simulink subsystem "Shrimple_6dof_parachute"  (R2025a)
settings: Solver=VariableStepAuto  StartTime=0.0  StopTime=10.0  RelTol=1e-3
undefined symbols (not defined in the file): Apogee_stop, BG0, Burnout_stop, COM_table, F, HG0, I, ignition_delay, include_turbulence, latlong0, launch_elevation, Light, m_table, MIL, MOI_table, time0, turbulence_noise_seeds, uvw0_B, v0_NED, w0_BN, x0_NED
libraries: sharedtransform x2, aerolibwind2 x1
settings Model: Creator=thatf  LastModifiedBy=thatf
settings RTWCC: GPUComputeCapability=3.5

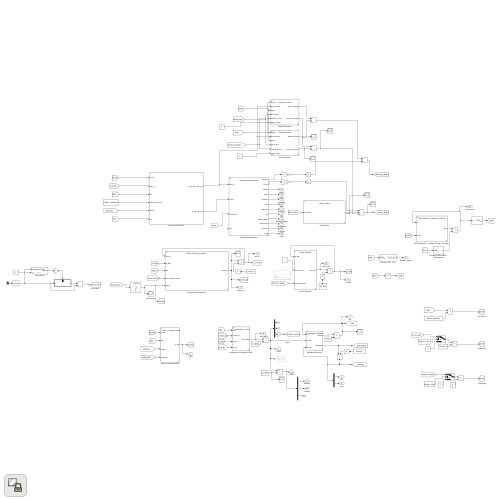
[thumbnail: Simulink's stored preview of the top-level diagram]
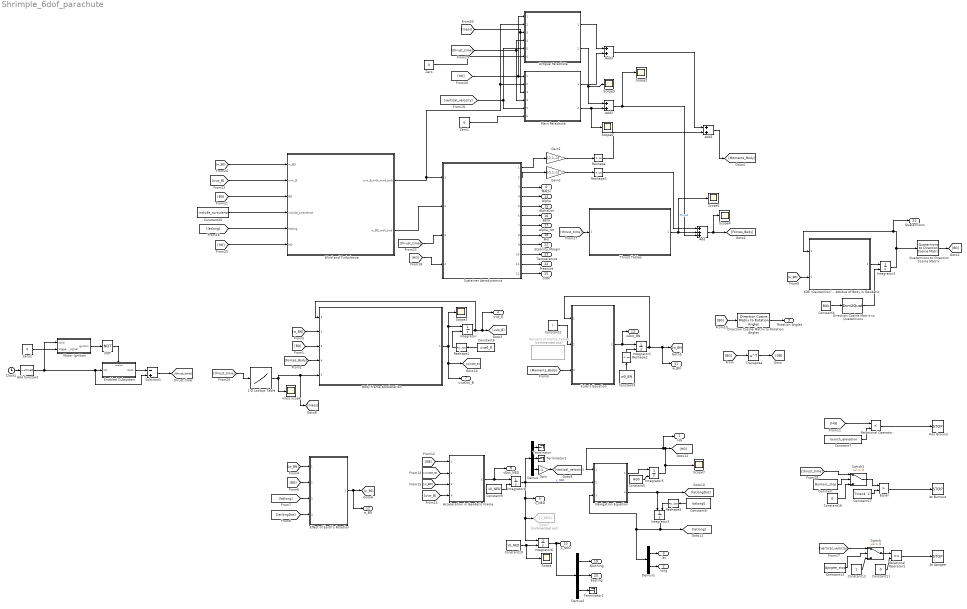
== system Shrimple_6dof_parachute ==
  1-D Lookup Table : Lookup_n-D  NumberOfTableDimensions=1  BreakpointsForDimension1=m_table(:,1)  Table=m_table(:,2)  InternalRulePriority=Speed  RndMeth=Simplest
  Acceleration in Geodetic Frame : Subsystem  ReferencedSubsystem=Acceleration_in_Geodetic_Frame
  Add : Sum  Inputs=+++
  Add Constant : Bias  Bias=time0  SaturateOnIntegerOverflow=off
  Add1 : Sum
  Add2 : Sum
  Add3 : Sum
  At Apogee : Stop
  At Burnout : Stop
  Body Frame Acceleration : Subsystem  ReferencedSubsystem=Body_Frame_Acceleration
  Clock1 : Clock
  Constant : Constant  Value=Burnout_stop
  Constant10 : Constant  Value=x0_NED
  Constant11 : Constant  Value=0
  Constant12 : Constant
  Constant13 : Constant  Value=Apogee_stop
  Constant16 : Constant  Value=0
  Constant17 : Constant  Value=Tx(end, 1)
  Constant2 : Constant  Value=I
  Constant20 : Constant  Value=include_turbulence
  Constant3 : Constant  Value=w0_BN
  Constant4 : Constant  Value=BG0
  Constant5 : Constant  Value=HG0
  Constant6 : Constant  Value=uvw0_B
  Constant7 : Constant  Value=launch_elevation
  Constant8 : Constant  Value=latlong0
  Constant9 : Constant  Value=v0_NED
  Demux : Demux  Outputs=3
  Demux1 : Demux  Outputs=2
  Demux2 : Demux  Outputs=3
  Direction Cosine Matrix to Rotation Angles : sharedtransform/Direction Cosine Matrix to Rotation Angles  rotationOrder=ZYX  aMode=aMode  action=None  tolerance=eps(2)
  Direction Cosine Matrix to Quaternions : Dcm2Quat
  Drogue Parachute : Subsystem  ReferencedSubsystem=Parachute_model  radius=drogue_radius  Cd=drogue_CD  parachute_deployment_type=ParachuteDeploymentType.Apogee_Delay_Deployment  burnout_delay=0  deploy_height=0
  Effect of Earth's Rotation : Subsystem  ReferencedSubsystem=Effect_of_Earths_Rotation
  Enabled Subsystem : Subsystem  TreatAsAtomicUnit=on
  Equal : RelationalOperator  Operator=>  OutDataTypeStr=boolean  RndMeth=Simplest  InputSameDT=off
  Euler's Equation : Subsystem  ReferencedSubsystem=Eulers_Equation
  Gain : Gain  Gain=-1
  Gain1 : Gain  Gain=[-1,1,-1]
  Gain2 : Gain  Gain=[-1,1,-1]
  Goto7 : Goto  Commented=on  GotoTag=v_NED
  Hits Ground : Stop
  Integrator{,1..6} (7 alike) : Integrator  InitialConditionSource=external
  "KDE (Qauternion) -  Attidue of Body in Geodetic " : Subsystem  ReferencedSubsystem=KDE_Qauternion_Attitude_of_Body_in_Geodetic
  Main Parachute : Subsystem  ReferencedSubsystem=Parachute_model  radius=main_radius  Cd=main_CD  parachute_deployment_type=ParachuteDeploymentType.Elevation_Deployment  burnout_delay=0  deploy_height=300
  Moment of Inertia Tables : Subsystem  Commented=on
  Motor Ignition : Subsystem  Variant=on
  NOT : Logic  Operator=NOT  IconShape=distinctive  AllPortsSameDT=off  OutDataTypeStr=boolean
  Navigation Equation : Subsystem  ReferencedSubsystem=Navigation_Equation
  Quaternions to Direction Cosine Matrix : sharedtransform/Quaternions to  Direction Cosine Matrix  aMode=aMode
  Relational Operator : RelationalOperator  Operator=<  OutDataTypeStr=boolean  RndMeth=Simplest  InputSameDT=off
  Relational Operator1 : RelationalOperator  Operator=<=  OutDataTypeStr=boolean  RndMeth=Simplest  InputSameDT=off
  Reshape{,1..3} (4 alike) : Reshape  OutputDimensionality=Customize  OutputDimensions=[3,1]
  Reshape4 : Reshape  OutputDimensionality=Customize  OutputDimensions=[2,1]
  Scope{,1..7} (8 alike) : Scope
      Scope settings: ActiveDisplayYMinimum=-435.13988  ActiveDisplayYMaximum=48.34887  DataLoggingVariableName=ScopeData11
      Scope1 settings: ActiveDisplayYMinimum=-123.17299  ActiveDisplayYMaximum=58.34227  DataLoggingVariableName=ScopeData12
      Scope2 settings: ActiveDisplayYMinimum=-1  ActiveDisplayYMaximum=1  DataLoggingVariableName=ScopeData13
      Scope3 settings: ActiveDisplayYMinimum=-153.18625  ActiveDisplayYMaximum=463.92065  DataLoggingVariableName=ScopeData14
      Scope4 settings: ActiveDisplayYMinimum=-123.17299  ActiveDisplayYMaximum=58.34227  DataLoggingVariableName=ScopeData15
      Scope5 settings: ActiveDisplayYMinimum=-1  ActiveDisplayYMaximum=1  DataLoggingVariableName=ScopeData7
      Scope6 settings: ActiveDisplayYMinimum=-1  ActiveDisplayYMaximum=1  DataLoggingVariableName=ScopeData8
      Scope7 settings: ActiveDisplayYMinimum=-1765.05046  ActiveDisplayYMaximum=15985.4541  DataLoggingVariableName=ScopeData16
  Subtract1 : Sum  Inputs=-+
  Sustainer Aerodynamics : Subsystem  ReferencedSubsystem=Sustainer_Aerodynamics
  Switch : Switch  Criteria=u2 > Threshold  SaturateOnIntegerOverflow=off  InputSameDT=off
  Switch1 : Switch  Criteria=u2 > Threshold  SaturateOnIntegerOverflow=off  InputSameDT=off
  Terminator : Terminator
  Terminator1 : Terminator
  Terminator2 : Terminator
  Thrust Tables : Subsystem  ReferencedSubsystem=Thrust_Tables
  Transpose : Math  Operator=transpose
  Wind and Turbulence : Subsystem
  Zero : Constant  Value=0  OutDataTypeStr=Inherit: Inherit via back propagation
  Zero1 : Constant  Value=0  OutDataTypeStr=Inherit: Inherit via back propagation
  Zero2 : Constant  Value=0  OutDataTypeStr=Inherit: Inherit via back propagation
  mass scope : Scope
      settings: ActiveDisplayYMinimum=12.9015  ActiveDisplayYMaximum=24.17549  DataLoggingVariableName=ScopeData17
  HG : Outport
  long : Outport  Port=2
  lat : Outport  Port=3
  uvw_B : Outport  Port=4
  v_NED : Outport  Port=5
  MACH : Outport  Port=6
  uvwDot_B : Outport  Port=7
  vDot_NED : Outport  Port=8
  Rotation Angles : Outport  Port=9
  x_NED : Outport  Port=10
  w_BN : Outport  Port=11
  w_BG : Outport  Port=12
  wDot_BN : Outport  Port=13
  Alpha : Outport  Port=14
  AlphaDot : Outport  Port=15
  Beta : Outport  Port=16
  Alpha_tot : Outport  Port=17
  PHI : Outport  Port=18
  Northing : Outport  Port=19
  Easting : Outport  Port=20
  Quaternions : Outport  Port=21
  Stability_Margin : Outport  Port=22
  Temperature : Outport  Port=23
  Pressure : Outport  Port=24
  COM : Outport  Port=25
  wires:
  Euler's Equation/1 -> Integrator1/1, wDot_BN/1
  Direction Cosine Matrix to Rotation Angles/1 -> Rotation Angles/1
  [BG] -> Direction Cosine Matrix to Rotation Angles/1
  Direction Cosine Matrix to Quaternions/1 -> Integrator2/2
  Constant5/1 -> Integrator5/2
  [BG] -> Transpose/1
  [BG] -> Body Frame Acceleration/3
  [w_BG] -> Acceleration in Geodetic Frame/3
  Reshape/1 -> Add1/2
  Constant6/1 -> Reshape1/1
  Navigation Equation/2 -> Integrator3/1, [latlongDot]
  Integrator2/1 -> Quaternions to Direction Cosine Matrix/1, "KDE (Qauternion) -  Attidue of Body in Geodetic "/1, Quaternions/1
  Constant3/1 -> Reshape2/1
  [BG] -> Effect of Earth's Rotation/2
  [uvw_B] -> Acceleration in Geodetic Frame/4
  [w_BG] -> "KDE (Qauternion) -  Attidue of Body in Geodetic "/2
  Reshape2/1 -> Integrator1/2
  Reshape1/1 -> Integrator/2
  Integrator3/1 -> Navigation Equation/3, Demux1/1, [latlong]
  Acceleration in Geodetic Frame/1 -> Integrator4/1, vDot_NED/1
  Body Frame Acceleration/1 -> Integrator/1, Scope3/1, [uvwDot_B], uvwDot_B/1
  Navigation Equation/1 -> Integrator5/1
  Constant4/1 -> Direction Cosine Matrix to Quaternions/1
  Integrator5/1 -> [HG], HG/1, Navigation Equation/1, Scope7/1
  "KDE (Qauternion) -  Attidue of Body in Geodetic "/1 -> Integrator2/1
  [Moments_Body] -> Euler's Equation/3
  [w_BN] -> Effect of Earth's Rotation/1
  Integrator4/1 -> v_NED/1, Goto7/1, Integrator6/1, Navigation Equation/2, Demux/1  "v_NED"
  [w_BN] -> Body Frame Acceleration/2
  Integrator/1 -> Body Frame Acceleration/1, [uvw_B], uvw_B/1
  Quaternions to Direction Cosine Matrix/1 -> [BG]
  [uvwDot_B] -> Acceleration in Geodetic Frame/2
  Effect of Earth's Rotation/1 -> [w_BG], w_BG/1
  [GB] -> Acceleration in Geodetic Frame/1
  Transpose/1 -> [GB]
  Relational Operator/1 -> Hits Ground/1
  [Forces_Body] -> Body Frame Acceleration/4
  [latlongDot] -> Effect of Earth's Rotation/4
  Constant7/1 -> Relational Operator/2
  [latlong] -> Effect of Earth's Rotation/3
  Constant9/1 -> Integrator4/2
  Reshape4/1 -> Integrator3/2
  Integrator1/1 -> Euler's Equation/1, [w_BN], w_BN/1
  Constant8/1 -> Reshape4/1
  Demux1/2 -> long/1
  Demux1/1 -> lat/1
  Constant10/1 -> Integrator6/2, Scope/1
  Integrator6/1 -> x_NED/1, Demux2/1
  Reshape3/1 -> Add/1
  Thrust Tables/1 -> Add/2, Scope1/1  "Thrust"
  Add/1 -> [Forces_Body], Scope4/1
  1-D Lookup Table/1 -> Body Frame Acceleration/5, [mass], mass scope/1
  Gain1/1 -> Reshape/1
  Gain2/1 -> Reshape3/1
  Demux2/3 -> Terminator2/1
  Sustainer Aerodynamics/8 -> PHI/1
  Sustainer Aerodynamics/7 -> Alpha_tot/1
  Sustainer Aerodynamics/6 -> Beta/1
  Sustainer Aerodynamics/5 -> AlphaDot/1
  Sustainer Aerodynamics/4 -> Alpha/1
  Sustainer Aerodynamics/3 -> MACH/1
  Sustainer Aerodynamics/2 -> Gain2/1
  Sustainer Aerodynamics/1 -> Gain1/1
  [HG] -> Sustainer Aerodynamics/4
  Sustainer Aerodynamics/9 -> Stability_Margin/1
  Equal/1 -> At Burnout/1
  Constant/1 -> Switch1/2
  Constant16/1 -> Switch1/3
  Constant17/1 -> Equal/2
  Switch1/1 -> Equal/1
  [thrust_time] -> Switch1/1
  Constant2/1 -> Euler's Equation/2
  Demux2/1 -> Northing/1
  Demux2/2 -> Easting/1
  [w_BG] -> Wind and Turbulence/1(w_BG)
  [uvw_B] -> Wind and Turbulence/2(uvw_B)
  [BG] -> Wind and Turbulence/3(BG)
  Constant20/1 -> Wind and Turbulence/4(include_turbulence)
  [latlong] -> Wind and Turbulence/5(latlong)
  [HG] -> Wind and Turbulence/6(HG)
  Wind and Turbulence/1(uvw_B_with_wind_turb) -> Sustainer Aerodynamics/1, Main Parachute/2, Drogue Parachute/2
  Wind and Turbulence/2(w_BG_with_turb) -> Sustainer Aerodynamics/2
  [HG] -> Relational Operator/1
  Constant13/1 -> Switch/2
  Constant12/1 -> Switch/3
  Switch/1 -> Relational Operator1/1
  Constant11/1 -> Relational Operator1/2
  Relational Operator1/1 -> At Apogee/1
  [HG] -> Main Parachute/1, Drogue Parachute/1
  [vertical_velocity] -> Drogue Parachute/5, Main Parachute/5
  Add1/1 -> [Moments_Body]
  Sustainer Aerodynamics/10 -> Temperature/1
  Sustainer Aerodynamics/11 -> Pressure/1
  Subtract1/1 -> [thrust_time]
  [thrust_time] -> 1-D Lookup Table/1
  [thrust_time] -> Thrust Tables/1
  Clock1/1 -> Add Constant/1
  Add Constant/1 -> Enabled Subsystem/1(In1), Subtract1/2, Motor Ignition/1(time)
  Enabled Subsystem/1(Out1) -> Subtract1/1
  Motor Ignition/1(ignition) -> NOT/1
  NOT/1 -> Enabled Subsystem/Enable
  [thrust_time] -> Drogue Parachute/4, Main Parachute/4
  [mass] -> Drogue Parachute/3, Main Parachute/3
  Add2/1 -> Add/3, Scope2/1
  Main Parachute/1 -> Add3/2
  Main Parachute/2 -> Add2/2, Scope6/1
  Add3/1 -> Add1/1
  Drogue Parachute/1 -> Add3/1
  Drogue Parachute/2 -> Add2/1, Scope5/1
  Demux/2 -> Terminator1/1
  Demux/1 -> Terminator/1
  Demux/3 -> Gain/1
  Gain/1 -> [vertical_velocity]
  [vertical_velocity] -> Switch/1
  Sustainer Aerodynamics/12 -> COM/1
  Zero/1 -> Drogue Parachute/6
  Zero1/1 -> Main Parachute/6
  Zero2/1 -> Motor Ignition/2(trigger_signal)
  [thrust_time] -> Sustainer Aerodynamics/3

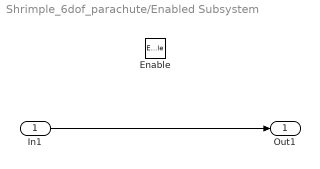
== system Shrimple_6dof_parachute/Enabled Subsystem ==
  In1 : Inport
  Enable : EnablePort
  Out1 : Outport
  wires:
  In1/1 -> Out1/1

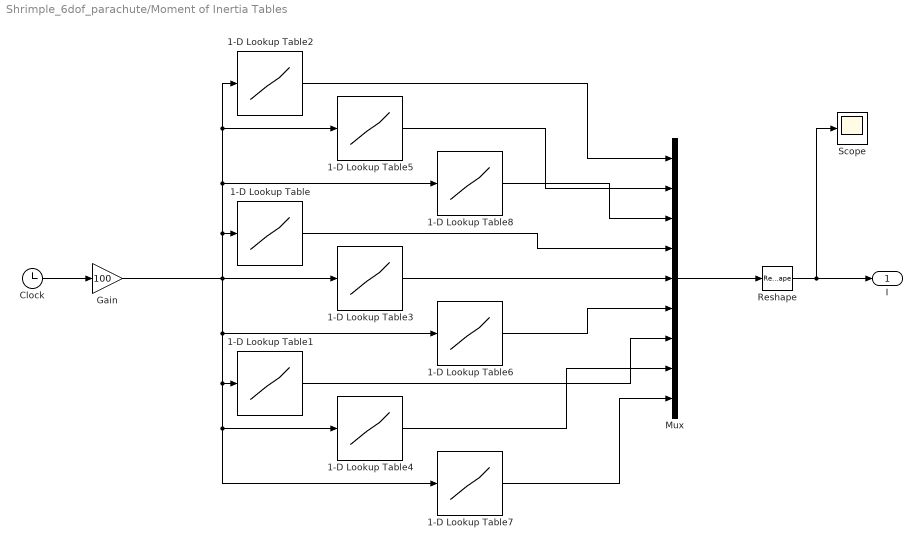
== system Shrimple_6dof_parachute/Moment of Inertia Tables ==
  1-D Lookup Table : Lookup_n-D  NumberOfTableDimensions=1  BreakpointsForDimension1=COM_table(:,1)  Table=MOI_table(:,2,1)  InternalRulePriority=Speed  RndMeth=Simplest
  1-D Lookup Table1 : Lookup_n-D  NumberOfTableDimensions=1  BreakpointsForDimension1=COM_table(:,1)  Table=MOI_table(:,3,1)  InternalRulePriority=Speed  RndMeth=Simplest
  1-D Lookup Table2 : Lookup_n-D  NumberOfTableDimensions=1  BreakpointsForDimension1=COM_table(:,1)  Table=MOI_table(:,1,1)  InternalRulePriority=Speed  RndMeth=Simplest
  1-D Lookup Table3 : Lookup_n-D  NumberOfTableDimensions=1  BreakpointsForDimension1=COM_table(:,1)  Table=MOI_table(:,2,2)  InternalRulePriority=Speed  RndMeth=Simplest
  1-D Lookup Table4 : Lookup_n-D  NumberOfTableDimensions=1  BreakpointsForDimension1=COM_table(:,1)  Table=MOI_table(:,3,2)  InternalRulePriority=Speed  RndMeth=Simplest
  1-D Lookup Table5 : Lookup_n-D  NumberOfTableDimensions=1  BreakpointsForDimension1=COM_table(:,1)  Table=MOI_table(:,1,2)  InternalRulePriority=Speed  RndMeth=Simplest
  1-D Lookup Table6 : Lookup_n-D  NumberOfTableDimensions=1  BreakpointsForDimension1=COM_table(:,1)  Table=MOI_table(:,2,3)  InternalRulePriority=Speed  RndMeth=Simplest
  1-D Lookup Table7 : Lookup_n-D  NumberOfTableDimensions=1  BreakpointsForDimension1=COM_table(:,1)  Table=MOI_table(:,3,3)  InternalRulePriority=Speed  RndMeth=Simplest
  1-D Lookup Table8 : Lookup_n-D  NumberOfTableDimensions=1  BreakpointsForDimension1=COM_table(:,1)  Table=MOI_table(:,1,3)  InternalRulePriority=Speed  RndMeth=Simplest
  Clock : Clock
  Gain : Gain  Gain=100
  Mux : Mux  Inputs=9
  Reshape : Reshape  OutputDimensionality=Customize  OutputDimensions=[3,3]
  Scope : Scope
      settings: ActiveDisplayYMinimum=-27.34629  ActiveDisplayYMaximum=20.83211  DataLoggingVariableName=ScopeData50
  I : Outport
  wires:
  Gain/1 -> 1-D Lookup Table6/1, 1-D Lookup Table1/1, 1-D Lookup Table4/1, 1-D Lookup Table7/1, 1-D Lookup Table3/1, 1-D Lookup Table/1, 1-D Lookup Table8/1, 1-D Lookup Table5/1, 1-D Lookup Table2/1
  Reshape/1 -> I/1, Scope/1
  Mux/1 -> Reshape/1
  1-D Lookup Table7/1 -> Mux/9
  1-D Lookup Table4/1 -> Mux/8
  1-D Lookup Table1/1 -> Mux/7
  1-D Lookup Table6/1 -> Mux/6
  1-D Lookup Table3/1 -> Mux/5
  1-D Lookup Table/1 -> Mux/4
  1-D Lookup Table8/1 -> Mux/3
  1-D Lookup Table5/1 -> Mux/2
  1-D Lookup Table2/1 -> Mux/1
  Clock/1 -> Gain/1

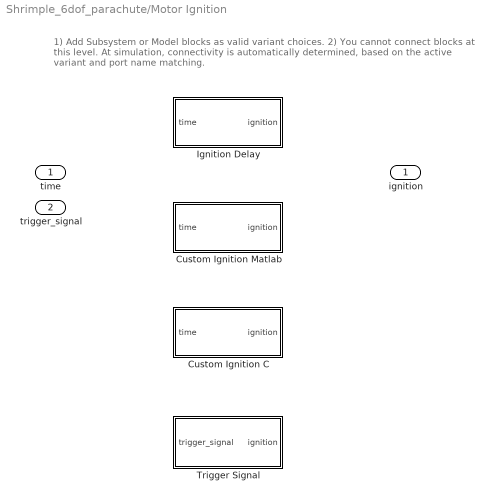
== system Shrimple_6dof_parachute/Motor Ignition ==
  note: 1) Add Subsystem or Model blocks as valid variant choices.
      | 2) You cannot connect blocks at this level. At simulation, connectivity is automatically
      | determined, based on the active variant and port name matching.
  time : Inport
  trigger_signal : Inport  Port=2
  Custom Ignition C : Subsystem  VariantControl=false
  Custom Ignition Matlab : Subsystem  VariantControl=false
  Ignition Delay : Subsystem  VariantControl=true
  Trigger Signal : Subsystem  VariantControl=false
  ignition : Outport

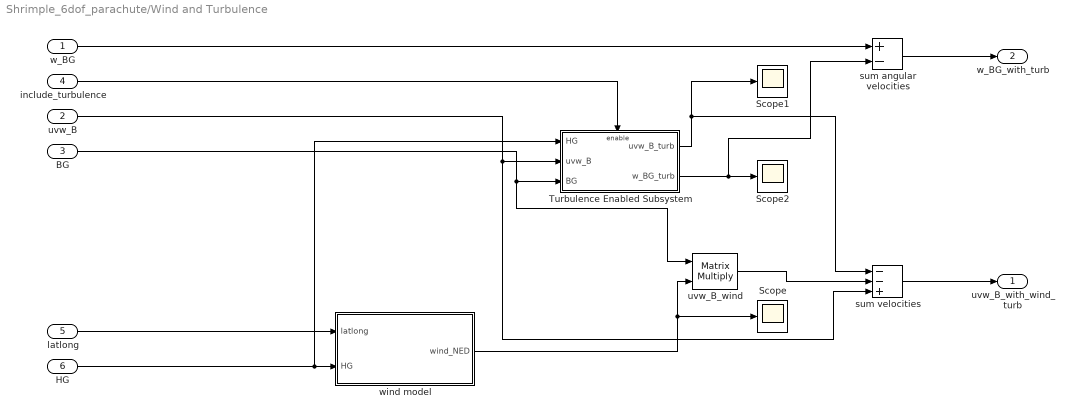
== system Shrimple_6dof_parachute/Wind and Turbulence ==
  w_BG : Inport
  uvw_B : Inport  Port=2
  BG : Inport  Port=3
  include_turbulence : Inport  Port=4
  latlong : Inport  Port=5
  HG : Inport  Port=6
  Scope : Scope
  Scope1 : Scope
  Scope2 : Scope
  Turbulence Enabled Subsystem : Subsystem  TreatAsAtomicUnit=on
  sum angular velocities : Sum  Inputs=+-
  sum velocities : Sum  Inputs=--+
  uvw_B_wind : Product  Multiplication=Matrix(*)
  wind model : Subsystem  Variant=on  VariantChoicesSpecifier={'Wind_Model_Systems/*.slx'}  VariantChoicesEnumeration=WindModelType  VariantControlVariable=wind_model_type
  uvw_B_with_wind_turb : Outport
  w_BG_with_turb : Outport  Port=2
  wires:
  Turbulence Enabled Subsystem/1(uvw_B_turb) -> sum velocities/1, Scope1/1
  Turbulence Enabled Subsystem/2(w_BG_turb) -> Scope2/1, sum angular velocities/2
  include_turbulence/1 -> Turbulence Enabled Subsystem/Enable
  sum velocities/1 -> uvw_B_with_wind_turb/1
  uvw_B_wind/1 -> sum velocities/2
  w_BG/1 -> sum angular velocities/1
  latlong/1 -> wind model/1(latlong)
  wind model/1(wind_NED) -> Scope/1, uvw_B_wind/2
  uvw_B/1 -> Turbulence Enabled Subsystem/2(uvw_B), sum velocities/3
  HG/1 -> Turbulence Enabled Subsystem/1(HG), wind model/2(HG)
  sum angular velocities/1 -> w_BG_with_turb/1
  BG/1 -> Turbulence Enabled Subsystem/3(BG), uvw_B_wind/1

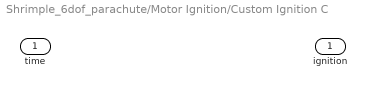
== system Shrimple_6dof_parachute/Motor Ignition/Custom Ignition C ==
  time : Inport
  ignition : Outport

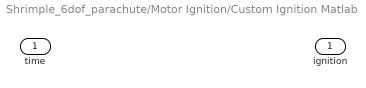
== system Shrimple_6dof_parachute/Motor Ignition/Custom Ignition Matlab ==
  time : Inport
  ignition : Outport

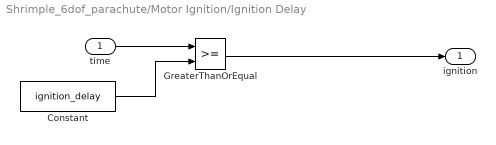
== system Shrimple_6dof_parachute/Motor Ignition/Ignition Delay ==
  time : Inport
  Constant : Constant  Value=ignition_delay
  GreaterThanOrEqual : RelationalOperator  OutDataTypeStr=boolean  RndMeth=Simplest  InputSameDT=off
  ignition : Outport
  wires:
  GreaterThanOrEqual/1 -> ignition/1
  Constant/1 -> GreaterThanOrEqual/2
  time/1 -> GreaterThanOrEqual/1

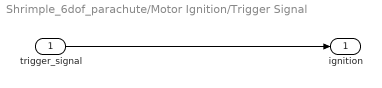
== system Shrimple_6dof_parachute/Motor Ignition/Trigger Signal ==
  trigger_signal : Inport
  ignition : Outport
  wires:
  trigger_signal/1 -> ignition/1

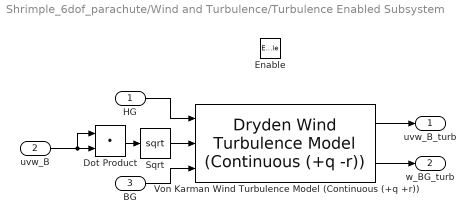
== system Shrimple_6dof_parachute/Wind and Turbulence/Turbulence Enabled Subsystem ==
  HG : Inport
  uvw_B : Inport  Port=2
  BG : Inport  Port=3
  Enable : EnablePort
  Dot Product : DotProduct  OutDataTypeStr=Inherit: Inherit via internal rule
  Sqrt : Sqrt
  Von Karman Wind Turbulence Model (Continuous (+q +r)) : aerolibwind2/Dryden Wind Turbulence Model  (Continuous (+q -r))  units=Metric (MKS)  spec=MIL-F-8785C  model=Continuous Von Karman (+q +r)  W20=wind_speed6m  Wdeg=wind_direction6m  TurbProb=10^-2 - Light  L_high=762  Wingspan=finspan  ts=0.1  Seed=turbulence_noise_seeds  T_on=on
      settings: LibrarySourceBlock=|
      | aerolibwind2/Von Karman Wind Turbulence Model
      | (Continuous (+q +r))
  uvw_B_turb : Outport
  w_BG_turb : Outport  Port=2
  wires:
  Von Karman Wind Turbulence Model (Continuous (+q +r))/2 -> w_BG_turb/1
  HG/1 -> Von Karman Wind Turbulence Model (Continuous (+q +r))/1
  Von Karman Wind Turbulence Model (Continuous (+q +r))/1 -> uvw_B_turb/1
  BG/1 -> Von Karman Wind Turbulence Model (Continuous (+q +r))/3
  Dot Product/1 -> Sqrt/1
  uvw_B/1 -> Dot Product/2, Dot Product/1
  Sqrt/1 -> Von Karman Wind Turbulence Model (Continuous (+q +r))/2

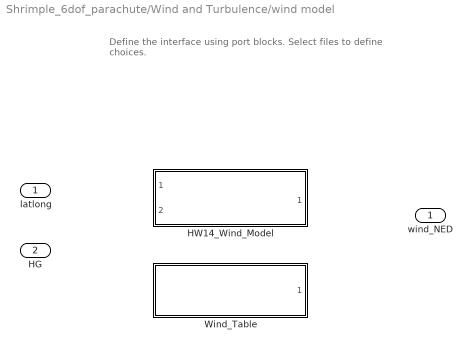
== system Shrimple_6dof_parachute/Wind and Turbulence/wind model ==
  note: Define the interface using port blocks.
      | Select files to define choices.
  latlong : Inport
  HG : Inport  Port=2
  HW14_Wind_Model : Subsystem  VariantControl=wind_model_type == WindModelType.HW14_Wind_Model  ReferencedSubsystem=HW14_Wind_Model
  Wind_Table : Subsystem  VariantControl=wind_model_type == WindModelType.Wind_Table  ReferencedSubsystem=Wind_Table
  wind_NED : Outport
